simulink model "lr6"  (R2022a)
settings: Solver=VariableStepAuto  StartTime=0.0  StopTime=20  RelTol=1e-3
libraries: instrumentseriallib x2
settings Model: Creator=User  LastModifiedBy=User

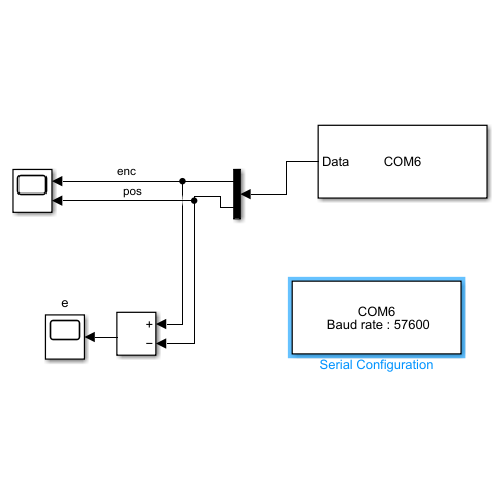
[thumbnail: Simulink's stored preview of the top-level diagram]
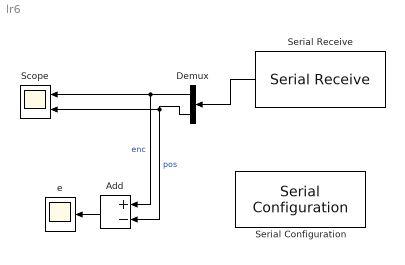
== system lr6 ==
  Add : Sum  Inputs=+-
  Demux : Demux  Outputs=2
  Scope : Scope  NumInputPorts=2
  Serial Configuration : instrumentseriallib/Serial Configuration  Priority=-200000  PortSel=COM6  Port=COM6  ComPort=COM6  BaudRate=57600  DataBits=8  Parity=none  StopBits=1  ByteOrder=little-endian  FlowControl=none  Timeout=3  SimulateUsing=Interpreted execution  BlockInModel=on  aMode=1
      settings: SourceProductBaseCode=OT,IC,MT
  Serial Receive : instrumentseriallib/Serial Receive  Priority=1  PortSel=COM6  Port=COM6  ComPort=COM6  DataType=int16  SaveDataType=uint8  ToggleHeader=on  Header='rrrr'  ToggleTerminator=on  Terminator=Custom terminator  CustomTerminator='nnnn'  InputFormat=Row major  ToggleDataSize=on  DataSize=[2]  EnableBlockingMode=on  ActionDataUnavailable=Output custom value  ActionWhenDataUnavailable=Output custom value  CustomValue=-1  SampleTime=0.01  SimulateUsing=Interpreted execution  BlockInModel=on  aMode=1
      settings: SourceProductBaseCode=OT,IC,MT
  e : Scope
  wires:
  Add/1 -> e/1
  Demux/1 -> Add/1, Scope/1  "enc"
  Serial Receive/1 -> Demux/1
  Demux/2 -> Scope/2, Add/2  "pos"
